simulink model "bandwidth_force"  (R2020b)
settings: Solver=ode4  StartTime=0.0  StopTime=10  FixedStep=1e-5  MaxStep=1e-4  RelTol=1e-4  EnableMultiTasking=on
values from neighbouring files (symbols this model uses):
  D = 0.1    [bandwidth.m]    (also in bandwidth_reference.m = 0.9; frequency_max_modulation_force.m = 0.9; frequency_max_modulation_force_sea.m = 0.9; frequency_max_modulation_position.m = 0.9)
  dm = 0.0068    [bandwidth.m]    (also in bandwidth_reference.m; frequency_max_modulation_force.m; frequency_max_modulation_force_sea.m; frequency_max_modulation_position.m)
  gear = 103    [bandwidth_reference.m]    (also in frequency_max_position.m; frequency_max_velocity.m; frequency_position.m; frequency_velocity.m)
  h = 100    [bandwidth_reference.m]    (also in force_control.m = h_vec(4); frequency_max_modulation_force.m = 2; frequency_max_modulation_force_sea.m = 10)
  Jm = 0.0064    [bandwidth.m]    (also in bandwidth_reference.m = 0.0104; frequency_max_modulation_force.m = 0.0104; frequency_max_modulation_force_sea.m = 0.0104; frequency_max_modulation_position.m = 0.0104)
  kt = 1.5038    [bandwidth_reference.m]    (also in frequency_max_modulation_force.m; frequency_max_modulation_force_sea.m; frequency_max_modulation_position.m; frequency_max_modulation_velocity.m)
  P = 15    [bandwidth.m]    (also in bandwidth_reference.m = 1; frequency_max_modulation_force.m = 10; frequency_max_modulation_force_sea.m = 10; frequency_max_modulation_position.m = 10)
settings Model: Creator=eldisondimo  LastModifiedBy=filippo
settings DataIOCC: LimitDataPoints=on  SaveOutput=off  SaveTime=off  ReturnWorkspaceOutputs=off
settings OptimizationCC: ExpressionDepthLimit=2147483647  LifeSpan=1
settings DebuggingCC: UnderspecifiedInitializationDetection=Classic  MergeDetectMultiDrivingBlocksExec=none  FcnCallInpInsideContextMsg=warning  AllowSymbolicDim=off  StateNameClashWarn=warning  SFUnexpectedBacktrackingDiag=warning  SFNoUnconditionalDefaultTransitionDiag=warning  SFExecutionAtInitializationDiag=none  ArithmeticOperatorsInVariantConditions=warning
settings SFSimCC: SimUseLocalCustomCode=off  CustomCodeUndefinedFunction=UseInterfaceOnly
settings RTWCC: RTWUseLocalCustomCode=off
settings CodeAppCC: StateflowObjectComments=on
settings GRTTargetCC: TargetLangStandard=C89/C90 (ANSI)  CombineOutputUpdateFcns=off  GRTInterface=on

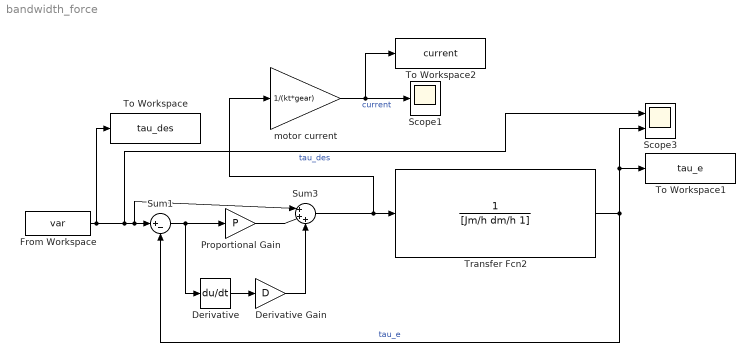
== system bandwidth_force ==
  Derivative : Derivative
  Derivative Gain : Gain  Gain=D
  From Workspace : FromWorkspace  VariableName=var
  Proportional Gain : Gain  Gain=P
  Scope1 : Scope
  Scope3 : Scope  NumInputPorts=2
  Sum1 : Sum  Inputs=|+-
  Sum3 : Sum  Inputs=|+++
  To Workspace : ToWorkspace  VariableName=tau_des  SaveFormat=Timeseries  SampleTime=-1
  To Workspace1 : ToWorkspace  VariableName=tau_e  SaveFormat=Timeseries  SampleTime=-1
  To Workspace2 : ToWorkspace  VariableName=current  SaveFormat=Timeseries  SampleTime=-1
  Transfer Fcn2 : TransferFcn  Denominator=[Jm/h dm/h 1]
  motor current : Gain  Gain=1/(kt*gear)
  wires:
  motor current/1 -> To Workspace2/1, Scope1/1  "current"
  Derivative/1 -> Derivative Gain/1
  Sum1/1 -> Derivative/1, Proportional Gain/1
  Sum3/1 -> Transfer Fcn2/1, motor current/1
  Transfer Fcn2/1 -> To Workspace1/1, Scope3/2, Sum1/2  "tau_e"
  From Workspace/1 -> To Workspace/1, Scope3/1, Sum3/1, Sum1/1  "tau_des"
  Proportional Gain/1 -> Sum3/2
  Derivative Gain/1 -> Sum3/3
